simulink model "register_file_lut"  (Simulink 7.4)
settings: Solver=ode45  StartTime=0.0  StopTime=500.0  RelTol=1e-3
values from neighbouring files (symbols this model uses):
  MAX_WARPS = 24    [register_file_lut.mat]
libraries: xbsIndex_r4 x17, simulink x1
settings Model: Creator=andryc  LastModifiedBy=andryc

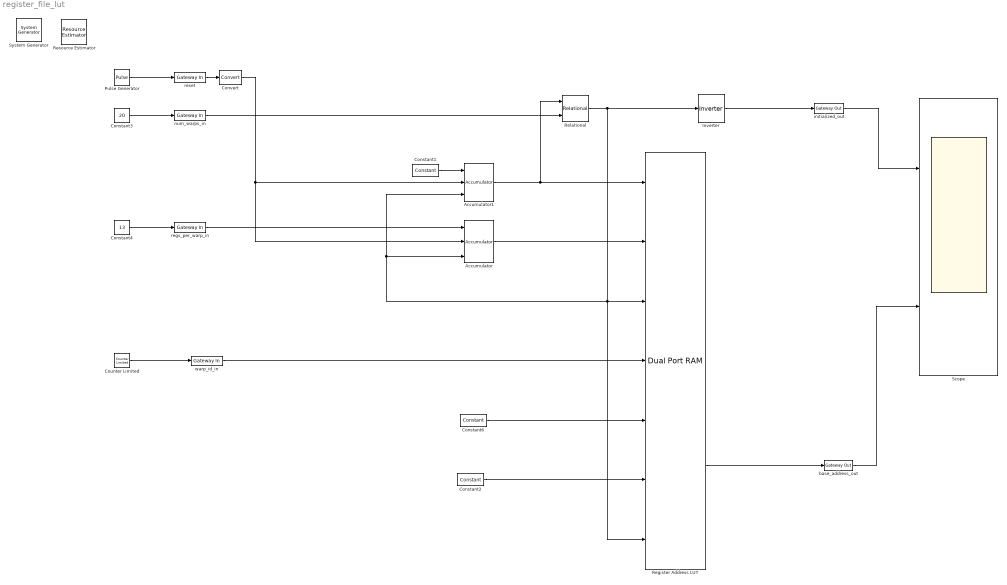
== system register_file_lut ==
  " System Generator" : xbsIndex_r4/ System Generator  Tag=genX  SystemSampleTime=-1  xilinxfamily=virtex5  part=xc5vlx50t  speed=-1  package=ff1136  synthesis_tool=XST  clock_wrapper=Clock Enables  directory=./ngc_netlist  testbench=off  simulink_period=1  sysclk_period=10  dcm_input_clock_period=10  incr_netlist=off  trim_vbits=Everywhere in SubSystem  dbl_ovrd=According to Block Masks  core_generation=According to Block Masks  run_coregen=off  deprecated_control=off  eval_field=0  block_type=sysgen
      settings: block_version=12.2
  Accumulator : xbsIndex_r4/Accumulator  operation=Add  n_bits=32  overflow=Wrap  scale=1  rst=on  hasbypass=off  en=on  dbl_ovrd=off  use_behavioral_HDL=on  implementation=Fabric  block_type=accum
      settings: block_version=12.2
  Accumulator1 : xbsIndex_r4/Accumulator  operation=Add  n_bits=5  overflow=Saturate  scale=1  rst=on  hasbypass=off  en=on  dbl_ovrd=off  use_behavioral_HDL=on  implementation=Fabric  block_type=accum
      settings: block_version=12.2
  Constant1 : xbsIndex_r4/Constant  arith_type=Unsigned  const=1  n_bits=9  bin_pt=0  explicit_period=off  period=1  equ=P=C  opselect=C  inp2=PCIN>>17  opr=+  inp1=P  carry=CIN  dbl_ovrd=off  block_type=constant
      settings: block_version=12.2
  Constant2 : xbsIndex_r4/Constant  arith_type=Boolean  const=0  n_bits=9  bin_pt=0  explicit_period=off  period=1  equ=P=C  opselect=C  inp2=PCIN>>17  opr=+  inp1=P  carry=CIN  dbl_ovrd=off  block_type=constant
      settings: block_version=12.2
  Constant3 : Constant  Value=20  OutDataType=fixdt(1, 16)  OutScaling=2^0
  Constant4 : Constant  Value=13  OutDataType=fixdt(1, 16)  OutScaling=2^0
  Constant6 : xbsIndex_r4/Constant  arith_type=Unsigned  const=0  n_bits=32  bin_pt=0  explicit_period=off  period=1  equ=P=C  opselect=C  inp2=PCIN>>17  opr=+  inp1=P  carry=CIN  dbl_ovrd=off  block_type=constant
      settings: block_version=12.2
  Convert : xbsIndex_r4/Convert  arith_type=Boolean  n_bits=16  bin_pt=14  quantization=Truncate  overflow=Wrap  en=off  latency=0  dbl_ovrd=off  pipeline=off  block_type=convert
      settings: block_version=12.2
  Counter Limited : simulink/Sources/Counter Limited  SystemSampleTime=-1  uplimit=20  tsamp=-1
  Inverter : xbsIndex_r4/Inverter  en=off  latency=0  dbl_ovrd=off  block_type=inv
      settings: block_version=12.2
  Pulse Generator : DiscretePulseGenerator  Amplitude=1  Period=500  PulseWidth=5  PhaseDelay=0  SampleTime=1
  Register Address LUT : xbsIndex_r4/Dual Port RAM  depth=MAX_WARPS+8  initVector=0  distributed_mem=Block RAM  init_a=0  init_b=0  rst_a=off  rst_b=off  en_a=on  en_b=off  latency=1  write_mode_A=Read After Write  write_mode_B=Read After Write  dbl_ovrd=off  optimize=Area  use_rpm=on  block_type=dpram
      settings: block_version=12.2
  Relational : xbsIndex_r4/Relational  mode=a<b  en=off  latency=0  dbl_ovrd=off  block_type=relational
      settings: block_version=12.2
  Resource Estimator : xbsIndex_r4/Resource Estimator  Tag=resEstTag  Slices=0  FFs=0  BRAMs=0  LUTs=0  IOBs=0  EBMs=0  TBUFs=0  xl_use_estimator_area=off  est_options=Estimate  block_type=resource_estimator
      settings: AttributesFormatString=Resource\nEstimator  block_version=12.2
  Scope : Scope  NumInputPorts=2
      settings: YMin=-5~-5  YMax=5~5
  base_address_out : xbsIndex_r4/Gateway Out  hdl_port=on  timing_constraint=None  locs_specified=off  LOCs={}  block_type=gatewayout
      settings: infoedit="Gateway out block.  Converts Xilinx fixed point inputs into ouputs of type Simulink integer, double, or fixed point.<br><br>Hardware notes:  In hardware these blocks become top level output ports or are discarded, depending on how they are configured."  block_version=12.2
  initialized_out : xbsIndex_r4/Gateway Out  hdl_port=on  timing_constraint=None  locs_specified=off  LOCs={}  block_type=gatewayout
      settings: infoedit="Gateway out block.  Converts Xilinx fixed point inputs into ouputs of type Simulink integer, double, or fixed point.<br><br>Hardware notes:  In hardware these blocks become top level output ports or are discarded, depending on how they are configured."  block_version=12.2
  num_warps_in : xbsIndex_r4/Gateway In  arith_type=Unsigned  n_bits=5  bin_pt=0  quantization=Truncate  overflow=Saturate  period=1  dbl_ovrd=off  timing_constraint=None  locs_specified=off  LOCs={}  hdl_port=on  block_type=gatewayin
      settings: infoedit="Gateway in block.  Converts inputs of type Simulink integer, double and fixed point to  Xilinx fixed point type.<br><br>Hardware notes:  In hardware these blocks become top level input ports."  block_version=12.2
  regs_per_warp_in : xbsIndex_r4/Gateway In  arith_type=Unsigned  n_bits=9  bin_pt=0  quantization=Truncate  overflow=Saturate  period=1  dbl_ovrd=off  timing_constraint=None  locs_specified=off  LOCs={}  hdl_port=on  block_type=gatewayin
      settings: infoedit="Gateway in block.  Converts inputs of type Simulink integer, double and fixed point to  Xilinx fixed point type.<br><br>Hardware notes:  In hardware these blocks become top level input ports."  block_version=12.2
  reset : xbsIndex_r4/Gateway In  arith_type=Unsigned  n_bits=1  bin_pt=0  quantization=Truncate  overflow=Saturate  period=1  dbl_ovrd=off  timing_constraint=None  locs_specified=off  LOCs={}  hdl_port=on  block_type=gatewayin
      settings: infoedit="Gateway in block.  Converts inputs of type Simulink integer, double and fixed point to  Xilinx fixed point type.<br><br>Hardware notes:  In hardware these blocks become top level input ports."  block_version=12.2
  warp_id_in : xbsIndex_r4/Gateway In  arith_type=Unsigned  n_bits=5  bin_pt=0  quantization=Truncate  overflow=Saturate  period=1  dbl_ovrd=off  timing_constraint=None  locs_specified=off  LOCs={}  hdl_port=on  block_type=gatewayin
      settings: infoedit="Gateway in block.  Converts inputs of type Simulink integer, double and fixed point to  Xilinx fixed point type.<br><br>Hardware notes:  In hardware these blocks become top level input ports."  block_version=12.2
  wires:
  regs_per_warp_in/1 -> Accumulator/1
  Constant1/1 -> Accumulator1/1
  num_warps_in/1 -> Relational/2
  reset/1 -> Convert/1
  warp_id_in/1 -> Register Address LUT/4
  Constant2/1 -> Register Address LUT/6
  Register Address LUT/2 -> base_address_out/1
  Inverter/1 -> initialized_out/1
  Constant3/1 -> num_warps_in/1
  Constant4/1 -> regs_per_warp_in/1
  Counter Limited/1 -> warp_id_in/1
  Constant6/1 -> Register Address LUT/5
  Pulse Generator/1 -> reset/1
  Convert/1 -> Accumulator1/2, Accumulator/2
  Relational/1 -> Inverter/1, Register Address LUT/7, Register Address LUT/3, Accumulator1/3, Accumulator/3
  initialized_out/1 -> Scope/1
  base_address_out/1 -> Scope/2
  Accumulator1/1 -> Register Address LUT/1, Relational/1
  Accumulator/1 -> Register Address LUT/2
